simulink model "compexx"  (R2023a)
settings: Solver=VariableStepAuto  StartTime=0.0  StopTime=10.0  RelTol=1e-3
values from neighbouring files (symbols this model uses):
  Ts = 10e-3    (= 0.01)    [GetExperimentData.m]    (also in compex.m = 0.2)
settings Model: Creator=rhea_saber  LastModifiedBy=hugom
settings OptimizationCC: ReuseModelBlockBuffer=off

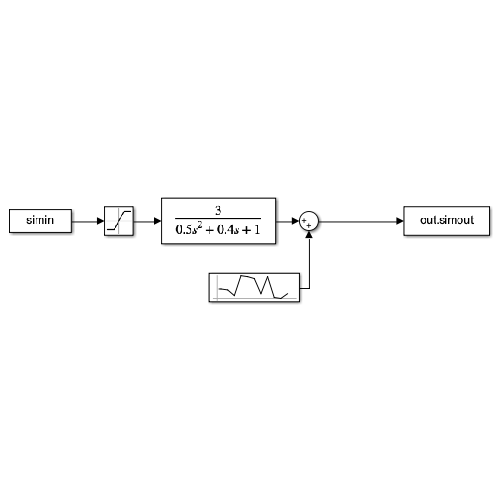
[thumbnail: Simulink's stored preview of the top-level diagram]
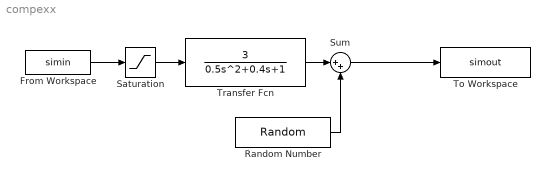
== system compexx ==
  From Workspace : FromWorkspace  VariableName=simin  SampleTime=Ts
  Random Number : RandomNumber  Variance=0.15  SampleTime=0.2
  Saturation : Saturate  UpperLimit=2  LowerLimit=-0.7  LinearizeAsGain=off  OutMin=-5  OutMax=5
  Sum : Sum  Inputs=|++
  To Workspace : ToWorkspace  VariableName=simout  SaveFormat=Structure With Time  SampleTime=Ts
  Transfer Fcn : TransferFcn  Numerator=[3]  Denominator=[0.5 0.4 1]
  wires:
  Transfer Fcn/1 -> Sum/1
  Sum/1 -> To Workspace/1
  Saturation/1 -> Transfer Fcn/1
  From Workspace/1 -> Saturation/1
  Random Number/1 -> Sum/2
